simulink model "less_conservative_algorithm_dc"  (R2015b)
settings: Solver=ode3  StartTime=0.0  StopTime=40  RelTol=1e-3
values from neighbouring files (symbols this model uses):
  bHI = 1    [Initiation.m]
  bWall = 0    [Initiation.m]    (also in VirtualEnvironment.m = diag(block.DialogPrm(2).Data))
  cSphere = [0; 0; 0]    [Initiation.m]
  direction = [0; 0; -1]    [Initiation.m]
  F_hand = 10    [Initiation.m]
  kWall = 1000000    [Initiation.m]    (also in VirtualEnvironment.m = diag(block.DialogPrm(1).Data))
  m = 1    [Initiation.m]
  nWall = 1    [Initiation.m]    (also in VirtualEnvironment.m = block.DialogPrm(3).Data)
  p0 = [0;0;15]    [Initiation.m]    (also in controller2.m = block.DialogPrm(4).Data)
  tsampling = block.DialogPrm(3).Data    [Controller.m]    (also in Controller_more.m = block.DialogPrm(4).Data; Initiation.m = 0.001; VirtualEnvironment.m = block.DialogPrm(7).Data; controller2.m)
  v0 = [0;0;0]    [Initiation.m]    (also in Parameters.m = [0;0])
  xWall = 10    [Initiation.m]
libraries: simulink x2
settings Model: Creator=TOSHIBA  LastModifiedBy=TOSHIBA
settings DataIOCC: LimitDataPoints=off  SaveFormat=Array
settings HardwareCC: ProdWordSize=32  ProdHWDeviceType=Specified
settings GRTTargetCC: GeneratePreprocessorConditionals=Disable all

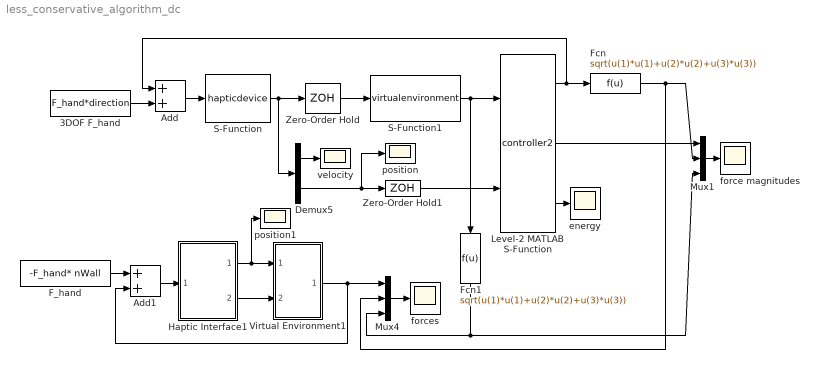
== system less_conservative_algorithm_dc ==
  3DOF F_hand : Constant  Value=F_hand*direction
  Add : Sum
  Add1 : Sum
  Demux5 : Demux  Outputs=2
  F_hand : Constant  Value=-F_hand* nWall
  Fcn : Fcn  Expr=sqrt(u(1)*u(1)+u(2)*u(2)+u(3)*u(3))
  Fcn1 : Fcn  Expr=sqrt(u(1)*u(1)+u(2)*u(2)+u(3)*u(3))
  Haptic Interface1 : Subsystem
  Level-2 MATLAB S-Function : M-S-Function  FunctionName=controller2  Parameters=dof, bHI, tsampling, p0
  Mux1 : Mux  Inputs=3
  Mux4 : Mux  Inputs=3
  S-Function : S-Function  FunctionName=hapticdevice  Parameters=m,bHI,v0,p0  SFunctionDeploymentMode=off  EnableBusSupport=off
  S-Function1 : S-Function  FunctionName=virtualenvironment  Parameters=kWall,bWall,xWall,cSphere  SFunctionDeploymentMode=off  EnableBusSupport=off
  Virtual Environment1 : Subsystem
  Zero-Order Hold : ZeroOrderHold  SampleTime=tsampling
  Zero-Order Hold1 : ZeroOrderHold  SampleTime=tsampling
  energy : Scope
  force magnitudes : Scope
  forces : Scope
  position : Scope
  position1 : Scope
  velocity : Scope
  wires:
  Add/1 -> S-Function/1
  S-Function/1 -> Demux5/1, Zero-Order Hold/1
  S-Function1/1 -> Fcn1/1, Level-2 MATLAB S-Function/1
  Haptic Interface1/2(Velocity) -> Virtual Environment1/2(velocity)
  Haptic Interface1/1(Position) -> position1/1, Virtual Environment1/1(position)
  Add1/1 -> Haptic Interface1/1(force)
  F_hand/1 -> Add1/1
  Virtual Environment1/1(fWall) -> Mux4/1, Add1/2
  Zero-Order Hold/1 -> S-Function1/1
  Mux4/1 -> forces/1
  Demux5/2 -> position/1, Zero-Order Hold1/1
  Demux5/1 -> velocity/1
  Level-2 MATLAB S-Function/1 -> Fcn/1, Add/1
  Level-2 MATLAB S-Function/3 -> energy/1
  3DOF F_hand/1 -> Add/2
  Zero-Order Hold1/1 -> Level-2 MATLAB S-Function/2
  Mux1/1 -> force magnitudes/1
  Level-2 MATLAB S-Function/2 -> Mux1/1
  Fcn/1 -> Mux4/2, Mux1/2
  Fcn1/1 -> Mux1/3, Mux4/3

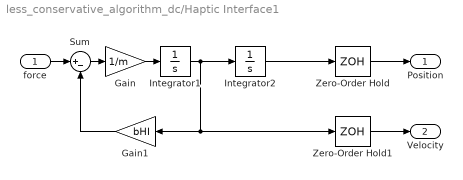
== system less_conservative_algorithm_dc/Haptic Interface1 ==
  force : Inport
  Gain : Gain  Gain=1/m
  Gain1 : Gain  Gain=bHI
  Integrator1 : Integrator  InitialCondition=v0(3)
  Integrator2 : Integrator  InitialCondition=p0(3)
  Sum : Sum  Inputs=|+-
  Zero-Order Hold : ZeroOrderHold  SampleTime=tsampling
  Zero-Order Hold1 : ZeroOrderHold  SampleTime=tsampling
  Position : Outport
  Velocity : Outport  Port=2
  wires:
  Integrator1/1 -> Zero-Order Hold1/1, Gain1/1, Integrator2/1
  Sum/1 -> Gain/1
  force/1 -> Sum/1
  Gain/1 -> Integrator1/1
  Gain1/1 -> Sum/2
  Integrator2/1 -> Zero-Order Hold/1
  Zero-Order Hold/1 -> Position/1
  Zero-Order Hold1/1 -> Velocity/1

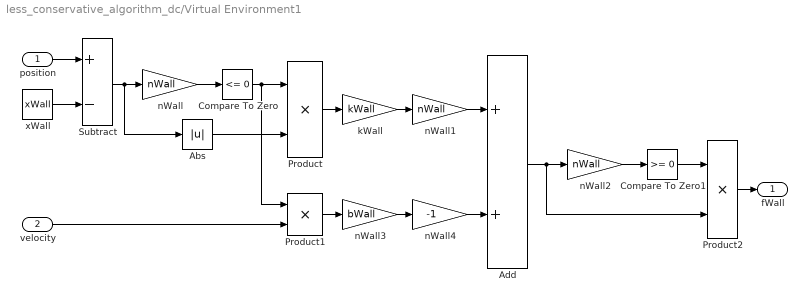
== system less_conservative_algorithm_dc/Virtual Environment1 ==
  position : Inport
  velocity : Inport  Port=2
  Abs : Abs
  Add : Sum
  Compare To Zero : simulink/Logic and Bit Operations/Compare To Zero  relop=<=  OutDataTypeStr=boolean
  Compare To Zero1 : simulink/Logic and Bit Operations/Compare To Zero  relop=>=  OutDataTypeStr=boolean
  Product : Product
  Product1 : Product
  Product2 : Product
  Subtract : Sum  Inputs=+-
  kWall : Gain  Gain=kWall
  nWall : Gain  Gain=nWall
  nWall1 : Gain  Gain=nWall
  nWall2 : Gain  Gain=nWall
  nWall3 : Gain  Gain=bWall
  nWall4 : Gain  Gain=-1
  xWall : Constant  Value=xWall
  fWall : Outport
  wires:
  Compare To Zero1/1 -> Product2/1
  nWall2/1 -> Compare To Zero1/1
  kWall/1 -> nWall1/1
  Product/1 -> kWall/1
  Abs/1 -> Product/2
  Compare To Zero/1 -> Product1/1, Product/1
  nWall/1 -> Compare To Zero/1
  Subtract/1 -> nWall/1, Abs/1
  position/1 -> Subtract/1
  xWall/1 -> Subtract/2
  nWall3/1 -> nWall4/1
  Product1/1 -> nWall3/1
  velocity/1 -> Product1/2
  nWall1/1 -> Add/1
  nWall4/1 -> Add/2
  Add/1 -> Product2/2, nWall2/1
  Product2/1 -> fWall/1
